simulink model "QuadSimulation"  (R2018b)
settings: Solver=VariableStepAuto  StartTime=0.0  StopTime=10.0  RelTol=1e-3
libraries: simulink x6, sharedutil x3, aerolibutil x3, vrlib x1
settings Model: Creator=soham  LastModifiedBy=soham

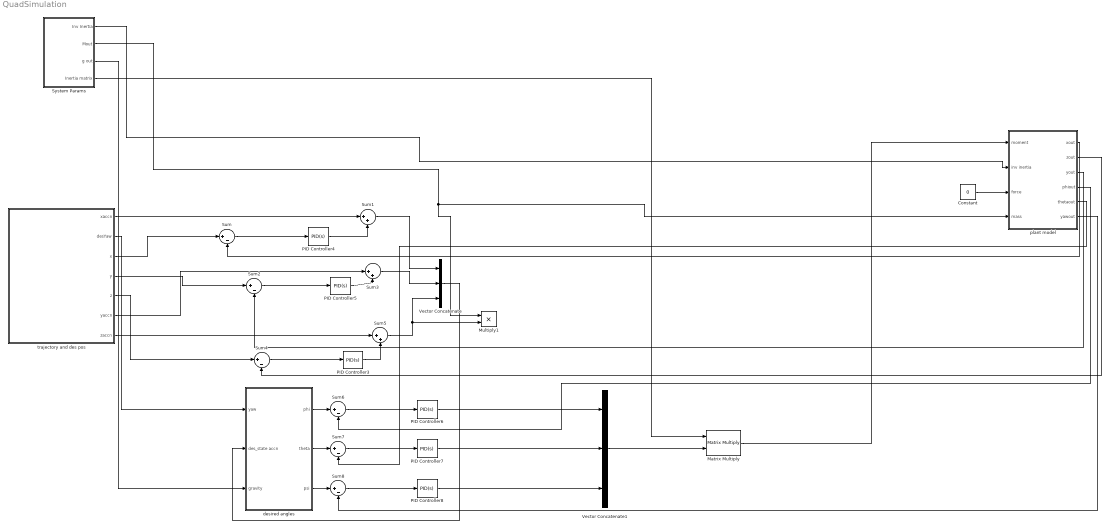
== system QuadSimulation ==
  Constant : Constant  Value=0
  Matrix Multiply : Product  Multiplication=Matrix(*)
  Multiply1 : Product
  PID Controller{3..8} (6 alike) : simulink/Continuous/PID Controller  Controller=PID  Form=Parallel  TimeDomain=Continuous-time  SampleTime=-1  IntegratorMethod=Forward Euler  FilterMethod=Forward Euler  ControllerParametersSource=internal  P=1  I=0  D=0  UseFilter=on  N=100  TunerSelectOption=Transfer Function Based (PID Tuner App)  InitialConditionSource=internal  InitialConditionForIntegrator=0  InitialConditionForFilter=0  DifferentiatorICPrevScaledInput=0  ExternalReset=none  TrackingMode=off  Kt=1  LimitOutput=off  UpperSaturationLimit=inf  LowerSaturationLimit=-inf  LinearizeAsGain=on  AntiWindupMode=none  Kb=1  POutMin=[]  POutMax=[]  IOutMin=[]  IOutMax=[]  DOutMin=[]  DOutMax=[]  NOutMin=[]  NOutMax=[]  SumOutMin=[]  SumOutMax=[]  SaturationOutMin=[]  SaturationOutMax=[]  PParamMin=[]  PParamMax=[]  IParamMin=[]  IParamMax=[]  DParamMin=[]  DParamMax=[]  NParamMin=[]  NParamMax=[]  KbParamMin=[]  KbParamMax=[]  KtParamMin=[]  KtParamMax=[]  KbOutMin=[]  KbOutMax=[]  KtOutMin=[]  KtOutMax=[]  IntegratorOutMin=[]  IntegratorOutMax=[]  FilterOutMin=[]  FilterOutMax=[]  SumI1OutMin=[]  SumI1OutMax=[]  SumI2OutMin=[]  SumI2OutMax=[]  SumI3OutMin=[]  SumI3OutMax=[]  SumI4OutMin=[]  SumI4OutMax=[]  SumDOutMin=[]  SumDOutMax=[]  DifferentiatorOutMin=[]  DifferentiatorOutMax=[]  FilterDiffOutCoefMin=[]  FilterDiffOutCoefMax=[]  ReciprocalOutMin=[]  ReciprocalOutMax=[]  SumDenOutMin=[]  SumDenOutMax=[]  SumNumOutMin=[]  SumNumOutMax=[]  DivideOutMin=[]  DivideOutMax=[]  IntegratorContinuousStateAttributes=''  IntegratorStateMustResolveToSignalObject=off  IntegratorRTWStateStorageClass=Auto  FilterContinuousStateAttributes=''  FilterStateMustResolveToSignalObject=off  FilterRTWStateStorageClass=Auto  ParallelPVariant=InternalParameters  IdealPVariant=Disabled  IVariant=InternalParameters  DVariant=InternalParameters  IntegratorVariant=Continuous  SatVariant=Disabled  AWVariant=Passthrough  PCopyVariant=Disabled  TRVariant=Disabled  FdbkBlocksVariant=Forward  IdealPFdbkVariant=Disabled  SatFdbkVariant=Disabled  DerivativeFilterVariant=ContFilter  NVariant=InternalParameters  NCopyVariant=Disabled  FilterICVariant=InternalICsFilter  IntegratorICVariant=InternalICs  ExternalResetVariant=Disabled  TRSumVariant=Passthrough  SumFdbkVariant=Disabled  SumVariant=Sum_PID
  Sum{,2,4,6..8} (6 alike) : Sum  Inputs=|+-
  Sum1 : Sum  Inputs=|++
  Sum3 : Sum  Inputs=|++
  Sum5 : Sum  Inputs=|++
  "System Params " : Subsystem
  Vector Concatenate : Concatenate  NumInputs=3  Mode=Multidimensional array
  Vector Concatenate1 : Concatenate  NumInputs=3  Mode=Multidimensional array
  "desired angles " : Subsystem
  "plant model " : Subsystem
  "trajectory and des pos " : Subsystem
  wires:
  "System Params "/2("Mout ") -> Multiply1/1, "plant model "/4("mass ")
  "System Params "/1("Inv Inertia ") -> "plant model "/2("inv inertia ")
  "plant model "/1("xout ") -> Sum/2
  Sum/1 -> PID Controller4/1
  "trajectory and des pos "/3("x ") -> Sum/1
  "trajectory and des pos "/1("xaccn ") -> Sum1/1
  PID Controller4/1 -> Sum1/2
  PID Controller5/1 -> Sum3/2
  Sum2/1 -> PID Controller5/1
  "plant model "/3("yout ") -> Sum2/2
  "trajectory and des pos "/4("y ") -> Sum2/1
  "trajectory and des pos "/6("yaccn ") -> Sum3/1
  PID Controller3/1 -> Sum5/2
  Sum4/1 -> PID Controller3/1
  "trajectory and des pos "/5("z ") -> Sum4/1
  "plant model "/2("zout ") -> Sum4/2
  "trajectory and des pos "/7("zaccn ") -> Sum5/1
  "trajectory and des pos "/2(desYaw) -> "desired angles "/1(yaw)
  "System Params "/3("g out ") -> "desired angles "/3(gravity)
  Sum1/1 -> Vector Concatenate/1
  Sum3/1 -> Vector Concatenate/2
  Sum5/1 -> Multiply1/2, Vector Concatenate/3
  Vector Concatenate/1 -> "desired angles "/2("des_state accn ")
  Sum6/1 -> PID Controller6/1
  "desired angles "/1("phi ") -> Sum6/1
  "plant model "/4("phiout ") -> Sum6/2
  Sum7/1 -> PID Controller7/1
  "desired angles "/2("theta ") -> Sum7/1
  "plant model "/5("thetaout ") -> Sum7/2
  Sum8/1 -> PID Controller8/1
  "desired angles "/3("psi ") -> Sum8/1
  "plant model "/6("yawout ") -> Sum8/2
  PID Controller6/1 -> Vector Concatenate1/1
  PID Controller7/1 -> Vector Concatenate1/2
  PID Controller8/1 -> Vector Concatenate1/3
  Vector Concatenate1/1 -> Matrix Multiply/2
  "System Params "/4("Inertia matrix ") -> Matrix Multiply/1
  Matrix Multiply/1 -> "plant model "/1("moment ")
  Constant/1 -> "plant model "/3("force ")

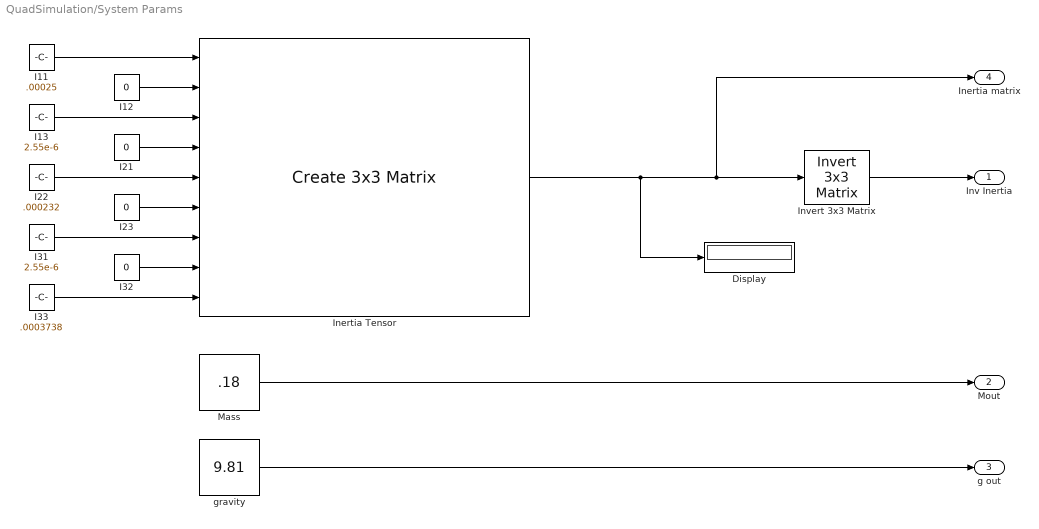
== system QuadSimulation/System Params  ==
  Display : Display
  I11 : Constant  Value=.00025
  I12 : Constant  Value=0
  "I13 " : Constant  Value=2.55e-6
  "I21 " : Constant  Value=0
  "I22 " : Constant  Value=.000232
  I23 : Constant  Value=0
  I31 : Constant  Value=2.55e-6
  I32 : Constant  Value=0
  "I33 " : Constant  Value=.0003738
  Inertia Tensor : sharedutil/Create 3x3 Matrix  aMode=aMode
  Invert 3x3 Matrix : aerolibutil/Invert  3x3 Matrix
  "Mass " : Constant  Value=.18
  gravity : Constant  Value=9.81
  "Inv Inertia " : Outport
  "Mout " : Outport  Port=2
  "g out " : Outport  Port=3
  "Inertia matrix " : Outport  Port=4
  wires:
  "I13 "/1 -> Inertia Tensor/3
  I32/1 -> Inertia Tensor/8
  "I22 "/1 -> Inertia Tensor/5
  Inertia Tensor/1 -> Display/1, "Inertia matrix "/1, Invert 3x3 Matrix/1
  "I33 "/1 -> Inertia Tensor/9
  Invert 3x3 Matrix/1 -> "Inv Inertia "/1
  I23/1 -> Inertia Tensor/6
  I31/1 -> Inertia Tensor/7
  "I21 "/1 -> Inertia Tensor/4
  I12/1 -> Inertia Tensor/2
  gravity/1 -> "g out "/1
  "Mass "/1 -> "Mout "/1
  I11/1 -> Inertia Tensor/1

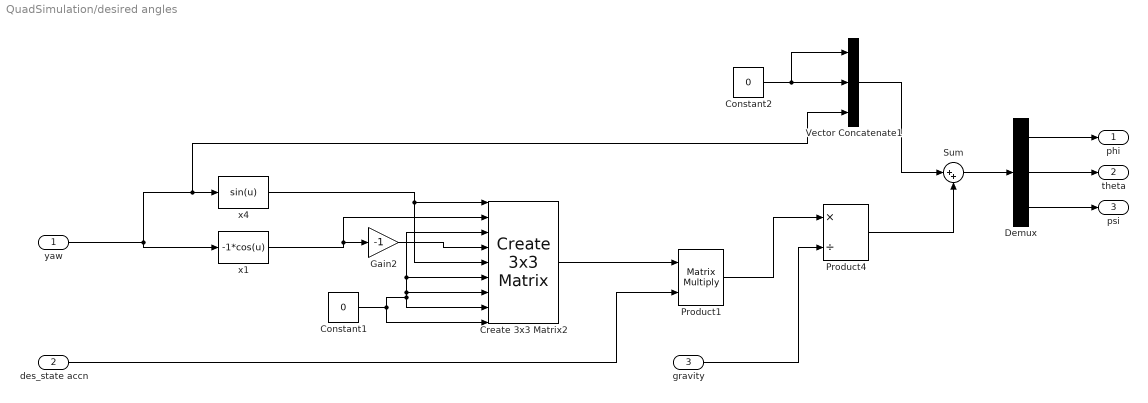
== system QuadSimulation/desired angles  ==
  yaw : Inport
  "des_state accn " : Inport  Port=2
  gravity : Inport  Port=3
  Constant1 : Constant  Value=0
  Constant2 : Constant  Value=0
  Create 3x3 Matrix2 : sharedutil/Create 3x3 Matrix  aMode=aMode
  Demux : Demux  Outputs=3
  Gain2 : Gain  Gain=-1
  Product1 : Product  Multiplication=Matrix(*)
  Product4 : Product  Inputs=*/
  Sum : Sum  Inputs=|++
  Vector Concatenate1 : Concatenate  NumInputs=3  Mode=Multidimensional array
  x1 : Fcn  Expr=-1*cos(u)
  x4 : Fcn  Expr=sin(u)
  "phi " : Outport
  "theta " : Outport  Port=2
  "psi " : Outport  Port=3
  wires:
  yaw/1 -> x1/1, Vector Concatenate1/3, x4/1
  "des_state accn "/1 -> Product1/2
  Product1/1 -> Product4/1
  Constant1/1 -> Create 3x3 Matrix2/8, Create 3x3 Matrix2/7, Create 3x3 Matrix2/6, Create 3x3 Matrix2/3, Create 3x3 Matrix2/9
  x4/1 -> Create 3x3 Matrix2/5, Create 3x3 Matrix2/1
  gravity/1 -> Product4/2
  Product4/1 -> Sum/2
  x1/1 -> Create 3x3 Matrix2/2, Gain2/1
  Vector Concatenate1/1 -> Sum/1
  Constant2/1 -> Vector Concatenate1/1, Vector Concatenate1/2
  Create 3x3 Matrix2/1 -> Product1/1
  Gain2/1 -> Create 3x3 Matrix2/4
  Sum/1 -> Demux/1
  Demux/3 -> "psi "/1
  Demux/2 -> "theta "/1
  Demux/1 -> "phi "/1

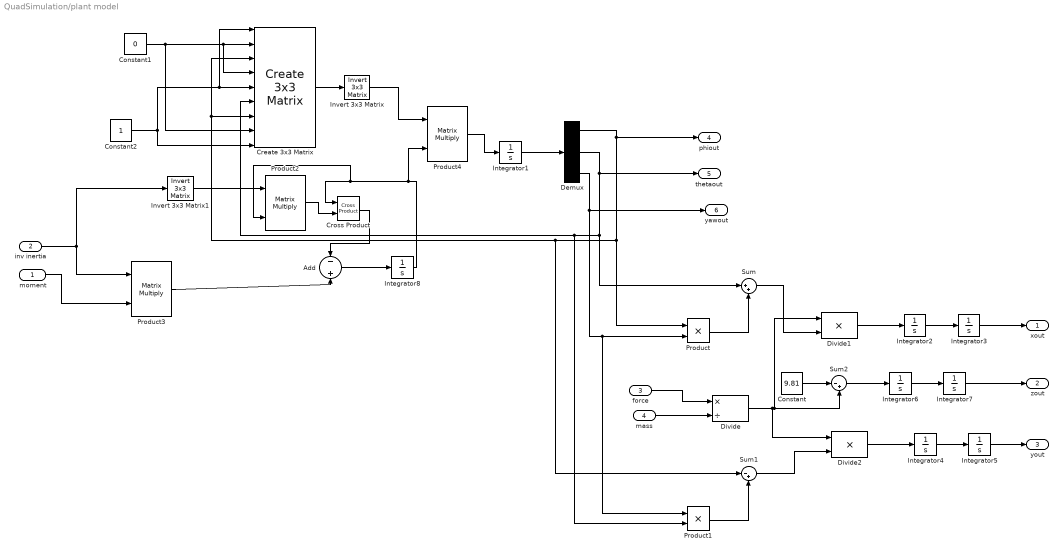
== system QuadSimulation/plant model  ==
  "moment " : Inport
  "inv inertia " : Inport  Port=2
  "force " : Inport  Port=3
  "mass " : Inport  Port=4
  Add : Sum  Inputs=-+
  Constant : Constant  Value=9.81
  Constant1 : Constant  Value=0
  Constant2 : Constant
  Create 3x3 Matrix : sharedutil/Create 3x3 Matrix  aMode=aMode
  Cross Product : vrlib/Utilities/Cross Product
      settings: SourceProductBaseCode=VR
  Demux : Demux  Outputs=3
  Divide : Product  Inputs=*/
  Divide1 : Product  Inputs=**
  Divide2 : Product  Inputs=**
  Integrator{1..8} (8 alike) : Integrator
  Invert 3x3 Matrix : aerolibutil/Invert  3x3 Matrix
  Invert 3x3 Matrix1 : aerolibutil/Invert  3x3 Matrix
  Product : Product
  Product1 : Product
  Product2 : Product  Multiplication=Matrix(*)
  Product3 : Product  Multiplication=Matrix(*)
  Product4 : Product  Multiplication=Matrix(*)
  Sum : Sum  Inputs=|++
  Sum1 : Sum  Inputs=|-+
  Sum2 : Sum  Inputs=|-+
  "xout " : Outport
  "zout " : Outport  Port=2
  "yout " : Outport  Port=3
  "phiout " : Outport  Port=4
  "thetaout " : Outport  Port=5
  "yawout " : Outport  Port=6
  wires:
  Integrator6/1 -> Integrator7/1
  Divide1/1 -> Integrator2/1
  Demux/1 -> "phiout "/1, Product/1, Sum1/1, Create 3x3 Matrix/3, Create 3x3 Matrix/7
  Demux/2 -> "thetaout "/1, Product1/2, Create 3x3 Matrix/6, Sum/1
  "mass "/1 -> Divide/2
  Integrator7/1 -> "zout "/1
  Product1/1 -> Sum1/2
  Constant2/1 -> Create 3x3 Matrix/1, Create 3x3 Matrix/5, Create 3x3 Matrix/9
  Integrator1/1 -> Demux/1
  Divide/1 -> Sum2/2, Divide1/1, Divide2/1
  Sum1/1 -> Divide2/2
  "inv inertia "/1 -> Invert 3x3 Matrix1/1, Product3/1
  Integrator5/1 -> "yout "/1
  Constant1/1 -> Create 3x3 Matrix/8, Create 3x3 Matrix/4, Create 3x3 Matrix/2
  Demux/3 -> "yawout "/1, Product1/1, Product/2
  Sum/1 -> Divide1/2
  Create 3x3 Matrix/1 -> Invert 3x3 Matrix/1
  Integrator3/1 -> "xout "/1
  Sum2/1 -> Integrator6/1
  "moment "/1 -> Product3/2
  Integrator4/1 -> Integrator5/1
  Product/1 -> Sum/2
  Divide2/1 -> Integrator4/1
  Constant/1 -> Sum2/1
  "force "/1 -> Divide/1
  Integrator2/1 -> Integrator3/1
  Invert 3x3 Matrix1/1 -> Product2/1
  Product3/1 -> Add/2
  Product2/1 -> Cross Product/2
  Cross Product/1 -> Add/1
  Add/1 -> Integrator8/1
  Integrator8/1 -> Product4/2, Product2/2, Cross Product/1
  Invert 3x3 Matrix/1 -> Product4/1
  Product4/1 -> Integrator1/1

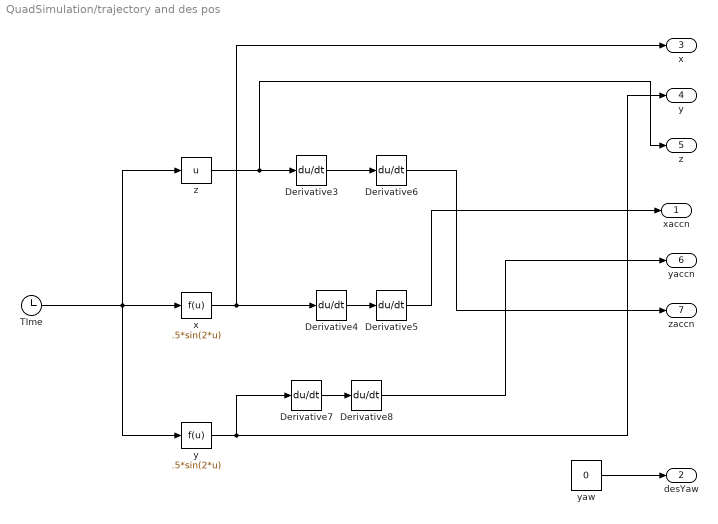
== system QuadSimulation/trajectory and des pos  ==
  Derivative{3..8} (6 alike) : Derivative
  "TIme " : Clock
  x : Fcn  Expr=.5*sin(2*u)
  y : Fcn  Expr=.5*sin(2*u)
  "yaw " : Constant  Value=0
  "z " : Fcn  Expr=u
  "xaccn " : Outport
  desYaw : Outport  Port=2
  "x " : Outport  Port=3
  "y " : Outport  Port=4
  "z " : Outport  Port=5
  "yaccn " : Outport  Port=6
  "zaccn " : Outport  Port=7
  wires:
  Derivative4/1 -> Derivative5/1
  "z "/1 -> "z "/1, Derivative3/1
  Derivative3/1 -> Derivative6/1
  Derivative8/1 -> "yaccn "/1
  x/1 -> "x "/1, Derivative4/1
  Derivative5/1 -> "xaccn "/1
  Derivative7/1 -> Derivative8/1
  "TIme "/1 -> "z "/1, y/1, x/1
  Derivative6/1 -> "zaccn "/1
  y/1 -> "y "/1, Derivative7/1
  "yaw "/1 -> desYaw/1
